simulink model "variation_luxIR_sim"  (R2024a)
settings: Solver=VariableStepAuto  StartTime=0.0  StopTime=50  RelTol=1e-3
PreLoadFcn:
  | params.NI0 = 0.1;      % LuxI初始密度
  | params.NR0 = 0.1;      % LuxR初始密度
  | params.A0 = 0;         % AHL初始浓度
  | params.rI = 0.7;       % LuxI生长速率
  | params.rR = 0.6;       % LuxR生长速率
  | params.K = 1.0;        % 环境承载力
  | params.kA = 0.1;       % AHL产生速率
  | params.dA = 0.05;      % AHL降解速率
  | params.delta = 0.01;   % 群体消耗系数
  | params.KA = 5;         % Hill阈值
  | params.n = 2;          % Hill系数
libraries: simulink x1
settings Model: Creator=22534  LastModifiedBy=22534

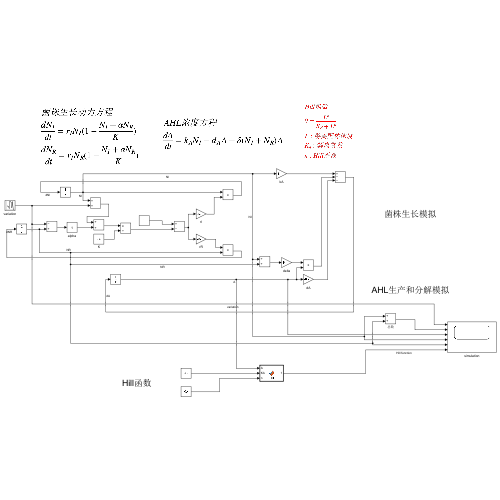
[thumbnail: Simulink's stored preview of the top-level diagram]
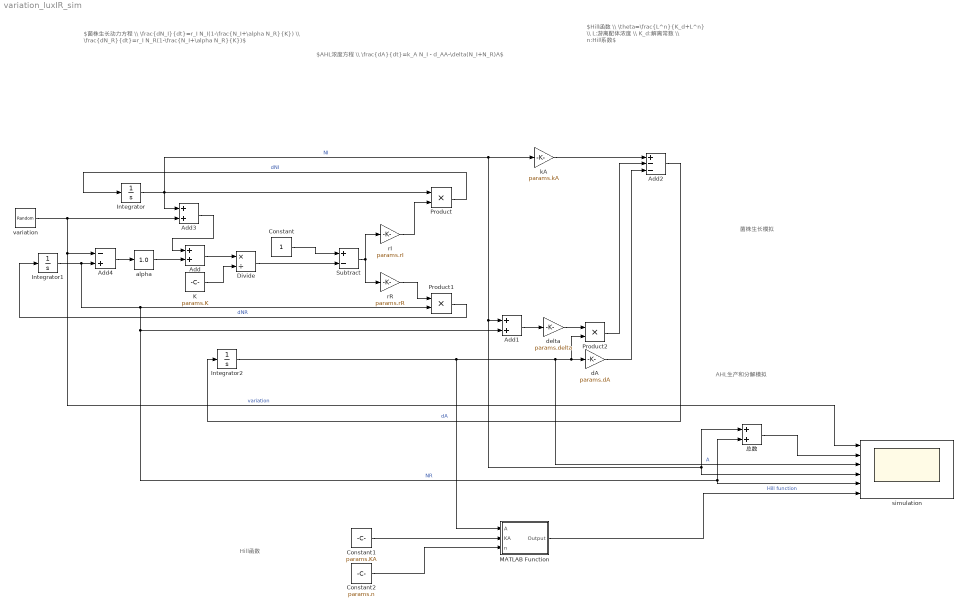
== system variation_luxIR_sim ==
  note: $Hill函数 \\ \theta=\frac{L^n}{K_d+L^n} \\ L:游离配体浓度 \\ K_d:解离常数 \\ n:Hill系数$
  note: 菌株生长模拟
  note: $菌株生长动力方程 \\ \frac{dN_I}{dt}=r_I N_I(1-\frac{N_I+\alpha N_R}{K}) \\ \frac{dN_R}{dt}=r_I N_R(1-\frac{N_I+\alpha N_R}{K})$
  note: $AHL浓度方程 \\ \frac{dA}{dt}=k_A N_I - d_AA-\delta(N_I+N_R)A$
  note: AHL生产和分解模拟
  note: Hill函数
  Add : Sum
  Add1 : Sum
  Add2 : Sum  Inputs=+--
  Add3 : Sum
  Add4 : Sum  Inputs=-+
  Constant : Constant
  Constant1 : Constant  Value=params.KA
  Constant2 : Constant  Value=params.n
  Divide : Product  Inputs=*/
  Integrator : Integrator  InitialCondition=params.NI0
  Integrator1 : Integrator  InitialCondition=params.NR0
  Integrator2 : Integrator  InitialCondition=params.A0
  K : Constant  Value=params.K
  MATLAB Function : MATLAB Function  TreatAsAtomicUnit=on
  Product : Product
  Product1 : Product
  Product2 : Product
  Subtract : Sum  Inputs=+-
  alpha : simulink/Math Operations/Slider Gain  gain=1.0  low=0  high=2
  dA : Gain  Gain=params.dA
  delta : Gain  Gain=params.delta
  kA : Gain  Gain=params.kA
  rI : Gain  Gain=params.rI
  rR : Gain  Gain=params.rR
  simulation : Scope  NumInputPorts=6
  variation : RandomNumber  Variance=0.01  SampleTime=0
  总数 : Sum
  wires:
  Integrator/1 -> Add3/1, 总数/1, simulation/4, Add1/1, kA/1, Product/1  "NI"
  Product/1 -> Integrator/1  "dNI"
  Integrator1/1 -> 总数/2, simulation/5, Add1/2, Product1/2, Add4/2  "NR"
  Product1/1 -> Integrator1/1  "dNR"
  Add/1 -> Divide/1
  K/1 -> Divide/2
  Constant/1 -> Subtract/1
  Divide/1 -> Subtract/2
  Subtract/1 -> rR/1, rI/1
  rI/1 -> Product/2
  rR/1 -> Product1/1
  alpha/1 -> Add/2
  Add2/1 -> Integrator2/1  "dA"
  Integrator2/1 -> simulation/3, dA/1, Product2/2, MATLAB Function/1(A)  "A"
  Add1/1 -> delta/1
  delta/1 -> Product2/1
  kA/1 -> Add2/1
  dA/1 -> Add2/3
  Product2/1 -> Add2/2
  Constant2/1 -> MATLAB Function/3(n)
  Constant1/1 -> MATLAB Function/2(KA)
  MATLAB Function/1(Output) -> simulation/6  "Hill function"
  variation/1 -> simulation/1, Add4/1, Add3/2  "variation"
  Add3/1 -> Add/1
  Add4/1 -> alpha/1
  总数/1 -> simulation/2

== matlab function variation_luxIR_sim/MATLAB Function ==
  data: A input; Output output; KA input; n input
function Output = Hill(A, KA, n)
   
Output = (A^n)/(KA^n+A^n);
